simulink model "ES238B_HwAgArbn"  (R2013b)
settings: Solver=ode45  StartTime=0.0  StopTime=10  FixedStep=.002  RelTol=1e-3
values from neighbouring files (symbols this model uses):
  HwAg = DataDict.OpSignal    [ES238B_HwAgArbn_DataDict.m]
  HWAGARBNMAXSTALL_CNT_U08 = DataDict.Constant    [ES238B_HwAgArbn_DataDict.m]
libraries: simulink x2
settings Model: RequirementInfo="{}  %GIDa_f9a11c6e_21fc_4cdc_9d0d_9c508fafadb2"  Creator=cz68ds  LastModifiedBy=CZ68DS
settings DebuggingCC: FrameProcessingCompatibilityMsg=error
settings GRTTargetCC: CodeReplacementLibrary=C89/C90 (ANSI)

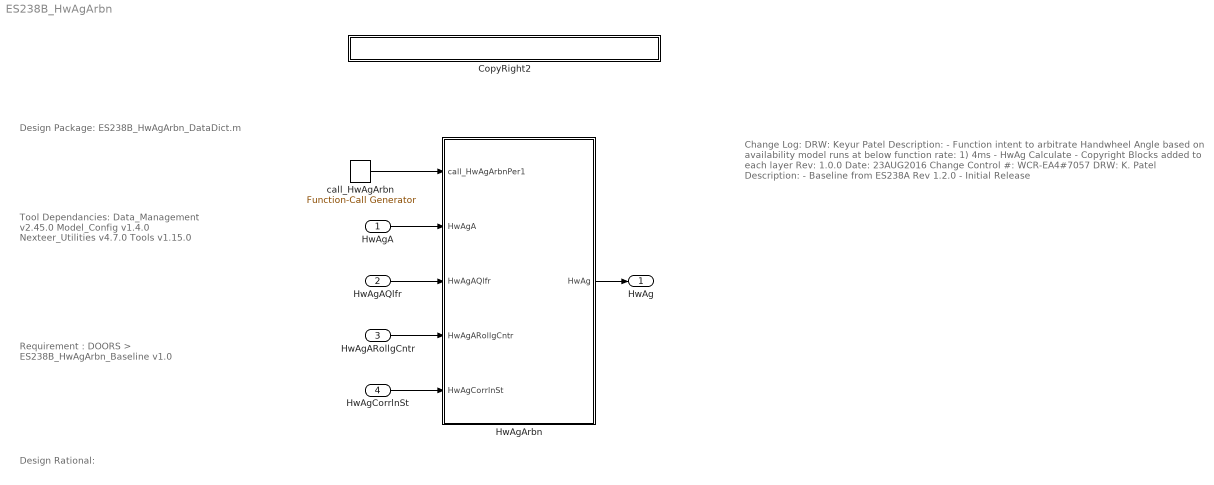
== system ES238B_HwAgArbn ==
  note: Design Package:
      |
      | ES238B_HwAgArbn_DataDict.m
  note: Tool Dependancies:
      |
      | Data_Management v2.45.0
      | Model_Config v1.4.0
      | Nexteer_Utilities v4.7.0
      | Tools v1.15.0
  note: Requirement :
      |
      | DOORS >
      | ES238B_HwAgArbn_Baseline v1.0
  note: Design Rational:
  note: Change Log:
      |
      | DRW: Keyur Patel
      | Description:
      | - Function intent to arbitrate Handwheel Angle based on availability
      |    model runs at below function rate:
      |       1) 4ms - HwAg Calculate
      | - Copyright Blocks added to each layer
      |
      | Rev: 1.0.0
      | Date: 23AUG2016
      | Change Control #: WCR-EA4#7057
      | DRW: K. Patel
      | Description:
      | - Baseline from ES238A Rev 1.2.0 - Initial Release
  HwAgA : Inport  OutDataTypeStr=single
  HwAgAQlfr : Inport  Port=2
  HwAgARollgCntr : Inport  Port=3
  HwAgCorrlnSt : Inport  Port=4
  CopyRight2 : Subsystem  Description=|  mask(Copyright Information){none=on}
      | Copyright info block.                                               
      |                                                                     
      | Place copyright information at the top of every subsystem in design.
      mask prompts: none "No parameters"
      mask help: Place copyright information at the top of every subsystem in design.
      mask Display:
      | NxtrConf = 'Nexteer Confidential';
      | 
      | sys = bdroot; %handle for the current model ("system")
      | first = get_param(sys,'Created');
      | first = first(end-3:end);  %year is last four digits
      | 
      | last = get_param(sys,'LastModifiedDate');
      | if isempty(last)
      |     last = datestr(now,'yyyy');
      | else
      |     last = last(end-3:end);
      | end
      | 
      | if strcmp(first,last)
      |     fprintf('%s -- Copyright %s Nexteer',NxtrConf,first)
      | else
      |     fprintf('%s -- %s%s- %s Nexteer',NxtrConf,char(169),first,last)
      | end
  HwAgArbn : Subsystem
      settings: AttributesFormatString=%<Tag>
  call_HwAgArbn : simulink/Ports & Subsystems/Function-Call Generator  sample_time=.004  numberOfIterations=1
      settings: AttributesFormatString=%<sample_time>
  HwAg : Outport
  wires:
  call_HwAgArbn/1 -> HwAgArbn/1(call_HwAgArbnPer1)
  HwAgA/1 -> HwAgArbn/2(HwAgA)
  HwAgAQlfr/1 -> HwAgArbn/3(HwAgAQlfr)
  HwAgARollgCntr/1 -> HwAgArbn/4(HwAgARollgCntr)
  HwAgCorrlnSt/1 -> HwAgArbn/5(HwAgCorrlnSt)
  HwAgArbn/1(HwAg) -> HwAg/1

== system ES238B_HwAgArbn/CopyRight2 ==

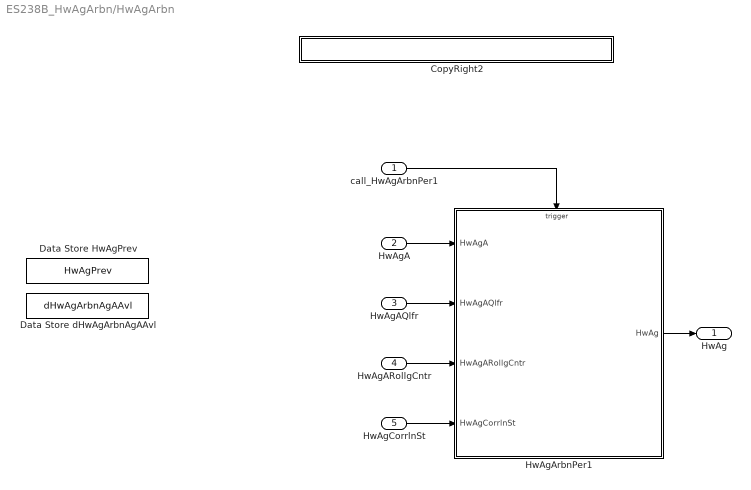
== system ES238B_HwAgArbn/HwAgArbn ==
  call_HwAgArbnPer1 : Inport
  HwAgA : Inport  Port=2  OutDataTypeStr=single
  HwAgAQlfr : Inport  Port=3
  HwAgARollgCntr : Inport  Port=4
  HwAgCorrlnSt : Inport  Port=5
  CopyRight2 : Subsystem  Description=|  mask(Copyright Information){none=on}
      | Copyright info block.                                               
      |                                                                     
      | Place copyright information at the top of every subsystem in design.
      mask prompts: none "No parameters"
      mask help: Place copyright information at the top of every subsystem in design.
      mask Display:
      | NxtrConf = 'Nexteer Confidential';
      | 
      | sys = bdroot; %handle for the current model ("system")
      | first = get_param(sys,'Created');
      | first = first(end-3:end);  %year is last four digits
      | 
      | last = get_param(sys,'LastModifiedDate');
      | if isempty(last)
      |     last = datestr(now,'yyyy');
      | else
      |     last = last(end-3:end);
      | end
      | 
      | if strcmp(first,last)
      |     fprintf('%s -- Copyright %s Nexteer',NxtrConf,first)
      | else
      |     fprintf('%s -- %s%s- %s Nexteer',NxtrConf,char(169),first,last)
      | end
  Data Store HwAgPrev : DataStoreMemory  DataStoreName=HwAgPrev  StateMustResolveToSignalObject=on
  Data Store dHwAgArbnAgAAvl : DataStoreMemory  DataStoreName=dHwAgArbnAgAAvl  StateMustResolveToSignalObject=on
  HwAgArbnPer1 : Subsystem  Tag=0.002  TreatAsAtomicUnit=on
  HwAg : Outport
  wires:
  call_HwAgArbnPer1/1 -> HwAgArbnPer1/Trigger
  HwAgAQlfr/1 -> HwAgArbnPer1/2(HwAgAQlfr)
  HwAgARollgCntr/1 -> HwAgArbnPer1/3(HwAgARollgCntr)
  HwAgArbnPer1/1(HwAg) -> HwAg/1
  HwAgA/1 -> HwAgArbnPer1/1(HwAgA)
  HwAgCorrlnSt/1 -> HwAgArbnPer1/4(HwAgCorrlnSt)

== system ES238B_HwAgArbn/HwAgArbn/CopyRight2 ==

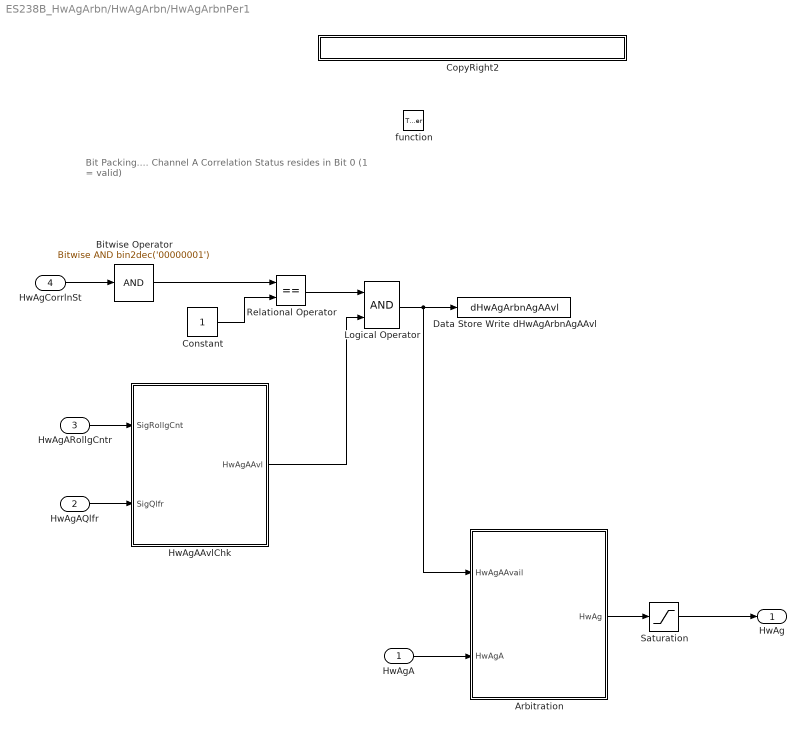
== system ES238B_HwAgArbn/HwAgArbn/HwAgArbnPer1 ==
  note: Bit Packing....
      | Channel A Correlation Status resides in Bit 0 (1 = valid)
  HwAgA : Inport
  HwAgAQlfr : Inport  Port=2
  HwAgARollgCntr : Inport  Port=3
  HwAgCorrlnSt : Inport  Port=4
  function : TriggerPort  TriggerType=function-call
  Arbitration : Subsystem  RequirementInfo={'linktype_rmi_doors' '00011b4b (/ESG Group/FDD Module Requirements/EA4 Specific/ES238B_HwAgArbn)' '#ES238B_21' 'true' 'REQ:ES238B_21' '' } %GIDa_cc4f3c33_a720_4edf_b686_36d833be5f87
  Bitwise Operator : simulink/Logic and Bit Operations/Bitwise Operator  RequirementInfo={} %GIDa_bea3dfe8_bd46_4f20_9050_0a8791fa4549  logicop=AND  UseBitMask=on  BitMask=bin2dec('00000001')  BitMaskRealWorld=Stored Integer
  Constant : Constant  RequirementInfo={} %GIDa_6ff7f489_96ba_46aa_b2f1_a64a9613b3ee  OutDataTypeStr=uint8
  CopyRight2 : Subsystem  Description=|  mask(Copyright Information){none=on}
      | Copyright info block.                                               
      |                                                                     
      | Place copyright information at the top of every subsystem in design.
      mask prompts: none "No parameters"
      mask help: Place copyright information at the top of every subsystem in design.
      mask Display:
      | NxtrConf = 'Nexteer Confidential';
      | 
      | sys = bdroot; %handle for the current model ("system")
      | first = get_param(sys,'Created');
      | first = first(end-3:end);  %year is last four digits
      | 
      | last = get_param(sys,'LastModifiedDate');
      | if isempty(last)
      |     last = datestr(now,'yyyy');
      | else
      |     last = last(end-3:end);
      | end
      | 
      | if strcmp(first,last)
      |     fprintf('%s -- Copyright %s Nexteer',NxtrConf,first)
      | else
      |     fprintf('%s -- %s%s- %s Nexteer',NxtrConf,char(169),first,last)
      | end
  Data Store Write dHwAgArbnAgAAvl : DataStoreWrite  RequirementInfo={'linktype_rmi_doors' '00011b4b (/ESG Group/FDD Module Requirements/EA4 Specific/ES238B_HwAgArbn)' '#ES238B_20' 'true' 'REQ:ES238B_20' '' } %GIDa_4a819c58_0746_455a_ab53_9583dea2382a  DataStoreName=dHwAgArbnAgAAvl
  HwAgAAvlChk : Subsystem  RequirementInfo={} %GIDa_384c42cc_0ffd_45df_a9b6_fe81dd918992  TreatAsAtomicUnit=on
  Logical Operator : Logic  RequirementInfo={} %GIDa_74228a93_0199_43c7_a692_a5e35af96634  AllPortsSameDT=off  OutDataTypeStr=boolean
  Relational Operator : RelationalOperator  RequirementInfo={} %GIDa_a4dfbfe0_37fd_46a5_994f_5fd593b15e89  Operator===  OutDataTypeStr=boolean
  Saturation : Saturate  UpperLimit=HwAg.EngMax  LowerLimit=HwAg.EngMin
      settings: AttributesFormatString=|
      | %<UpperLimit>=900
      | %<LowerLimit>=-900
  HwAg : Outport
  wires:
  HwAgARollgCntr/1 -> HwAgAAvlChk/1(SigRollgCnt)
  HwAgAQlfr/1 -> HwAgAAvlChk/2(SigQlfr)
  HwAgA/1 -> Arbitration/2(HwAgA)
  HwAgCorrlnSt/1 -> Bitwise Operator/1
  Bitwise Operator/1 -> Relational Operator/1
  Constant/1 -> Relational Operator/2
  Relational Operator/1 -> Logical Operator/1
  Logical Operator/1 -> Arbitration/1(HwAgAAvail), Data Store Write dHwAgArbnAgAAvl/1
  HwAgAAvlChk/1(HwAgAAvl) -> Logical Operator/2
  Arbitration/1(HwAg) -> Saturation/1
  Saturation/1 -> HwAg/1

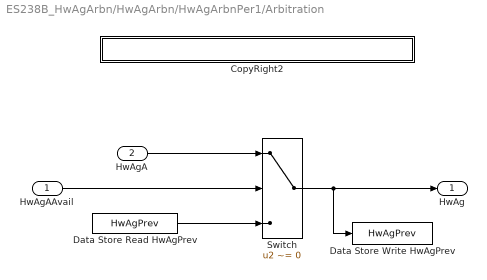
== system ES238B_HwAgArbn/HwAgArbn/HwAgArbnPer1/Arbitration ==
  HwAgAAvail : Inport
  HwAgA : Inport  Port=2
  CopyRight2 : Subsystem  Description=|  mask(Copyright Information){none=on}
      | Copyright info block.                                               
      |                                                                     
      | Place copyright information at the top of every subsystem in design.
      mask prompts: none "No parameters"
      mask help: Place copyright information at the top of every subsystem in design.
      mask Display:
      | NxtrConf = 'Nexteer Confidential';
      | 
      | sys = bdroot; %handle for the current model ("system")
      | first = get_param(sys,'Created');
      | first = first(end-3:end);  %year is last four digits
      | 
      | last = get_param(sys,'LastModifiedDate');
      | if isempty(last)
      |     last = datestr(now,'yyyy');
      | else
      |     last = last(end-3:end);
      | end
      | 
      | if strcmp(first,last)
      |     fprintf('%s -- Copyright %s Nexteer',NxtrConf,first)
      | else
      |     fprintf('%s -- %s%s- %s Nexteer',NxtrConf,char(169),first,last)
      | end
  Data Store Read HwAgPrev : DataStoreRead  DataStoreName=HwAgPrev
  Data Store Write HwAgPrev : DataStoreWrite  DataStoreName=HwAgPrev
  Switch : Switch  Criteria=u2 ~= 0
  HwAg : Outport
  wires:
  HwAgA/1 -> Switch/1
  HwAgAAvail/1 -> Switch/2
  Switch/1 -> Data Store Write HwAgPrev/1, HwAg/1
  Data Store Read HwAgPrev/1 -> Switch/3

== system ES238B_HwAgArbn/HwAgArbn/HwAgArbnPer1/CopyRight2 ==

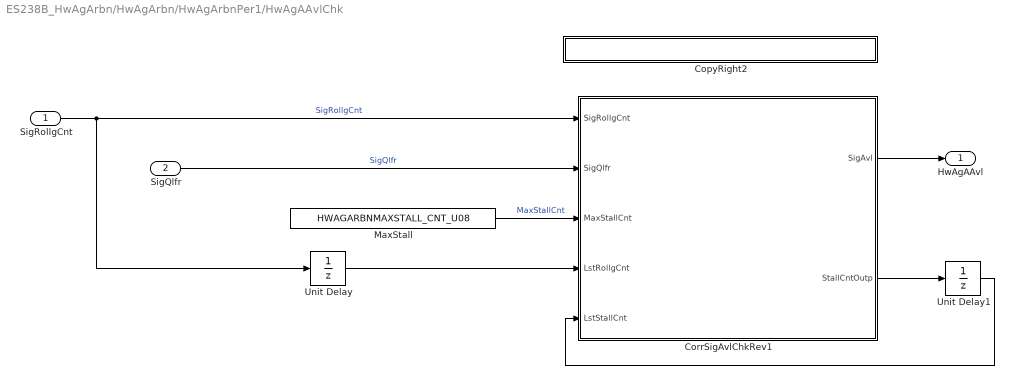
== system ES238B_HwAgArbn/HwAgArbn/HwAgArbnPer1/HwAgAAvlChk ==
  SigRollgCnt : Inport  OutDataTypeStr=uint8
  SigQlfr : Inport  Port=2  OutDataTypeStr=uint8
  CopyRight2 : Subsystem  Description=|  mask(Copyright Information){none=on}
      | Copyright info block.                                               
      |                                                                     
      | Place copyright information at the top of every subsystem in design.
      mask prompts: none "No parameters"
      mask help: Place copyright information at the top of every subsystem in design.
      mask Display:
      | NxtrConf = 'Nexteer Confidential';
      | 
      | sys = bdroot; %handle for the current model ("system")
      | first = get_param(sys,'Created');
      | first = first(end-3:end);  %year is last four digits
      | 
      | last = get_param(sys,'LastModifiedDate');
      | if isempty(last)
      |     last = datestr(now,'yyyy');
      | else
      |     last = last(end-3:end);
      | end
      | 
      | if strcmp(first,last)
      |     fprintf('%s -- Copyright %s Nexteer',NxtrConf,first)
      | else
      |     fprintf('%s -- %s%s- %s Nexteer',NxtrConf,char(169),first,last)
      | end
  CorrSigAvlChkRev1 : Stateflow chart  TreatAsAtomicUnit=on
  MaxStall : Constant  Value=HWAGARBNMAXSTALL_CNT_U08
  Unit Delay : UnitDelay  SampleTime=-1  StateName=HwAgARollgCntrPrev  StateMustResolveToSignalObject=on
      settings: AttributesFormatString=|
      | State Variable:
      | %<StateName>
  Unit Delay1 : UnitDelay  SampleTime=-1  StateName=HwAgAStallCntrPrev  StateMustResolveToSignalObject=on
      settings: AttributesFormatString=|
      | State Variable:
      | %<StateName>
  HwAgAAvl : Outport
  wires:
  SigRollgCnt/1 -> CorrSigAvlChkRev1/1(SigRollgCnt), Unit Delay/1  "SigRollgCnt"
  SigQlfr/1 -> CorrSigAvlChkRev1/2(SigQlfr)  "SigQlfr"
  MaxStall/1 -> CorrSigAvlChkRev1/3(MaxStallCnt)  "MaxStallCnt"
  Unit Delay/1 -> CorrSigAvlChkRev1/4(LstRollgCnt)
  CorrSigAvlChkRev1/2(StallCntOutp) -> Unit Delay1/1
  Unit Delay1/1 -> CorrSigAvlChkRev1/5(LstStallCnt)
  CorrSigAvlChkRev1/1(SigAvl) -> HwAgAAvl/1

== system ES238B_HwAgArbn/HwAgArbn/HwAgArbnPer1/Arbitration/CopyRight2 ==

== system ES238B_HwAgArbn/HwAgArbn/HwAgArbnPer1/HwAgAAvlChk/CopyRight2 ==

== stateflow chart ES238B_HwAgArbn/HwAgArbn/HwAgArbnPer1/HwAgAAvlChk/CorrSigAvlChkRev1 ==
  note: SigAvl
      | False = 0
      | Pass = 1
  note: SigQlfr
      | 0 = No Result
      | 1 = Pass
      | 2 = Fail
  (default) -> (junction 2)
  (junction 2) -> (junction 4) [order 1] : [SigRollgCnt ==LstRollgCnt]
  (junction 4) -> (junction 7) [order 2] : {
      | StallCntOutp = LstStallCnt +1;
      | }
  (junction 2) -> (junction 3) [order 2]
  (junction 4) -> (junction 7) [order 1] : [LstStallCnt == 255]
      | {
      | StallCntOutp = 255;
      | }
  (junction 3) -> (junction 7) : {
      | StallCntOutp = 0;
      | }
  (junction 7) -> (junction 10)
  (junction 10) -> (junction 12) [order 1] : [StallCntOutp >=MaxStallCnt]
  (junction 10) -> (junction 14) [order 2]
  (junction 12) -> (junction 17)
  (junction 14) -> (junction 17) [order 2]
  (junction 14) -> (junction 16) [order 1] : [SigQlfr<2]
  (junction 17) -> (junction 29) : {
      | SigAvl =0;
      | }
  (junction 16) -> (junction 29) : {
      | SigAvl = 1;
      | }
  data: SigRollgCnt input; SigQlfr input; MaxStallCnt input; SigAvl output uint8; LstRollgCnt input uint8; LstStallCnt input uint8; StallCntOutp output uint8
